simulink model "MCU_LPF_HPF"  (R2021b)
settings: Solver=FixedStepAuto  StartTime=0.0  StopTime=0.03  FixedStep=Ts  RelTol=1e-3
undefined symbols (not defined in the file): f_cutoff
libraries: simulink x1
settings Model: Creator=YeguKang  LastModifiedBy=qorgud1209
settings SFSimCC: SimCustomInitializer=init_software();  SimUserSources=microcontroller.c
settings SFSimCC: SimCustomHeaderCode=|
  | #include "microcontroller.h"
  | #include "Library/Software/headers/Filters.h"
  | #include "Library/Software/headers/ComplexFilters.h"
  | #include "Constants.h"

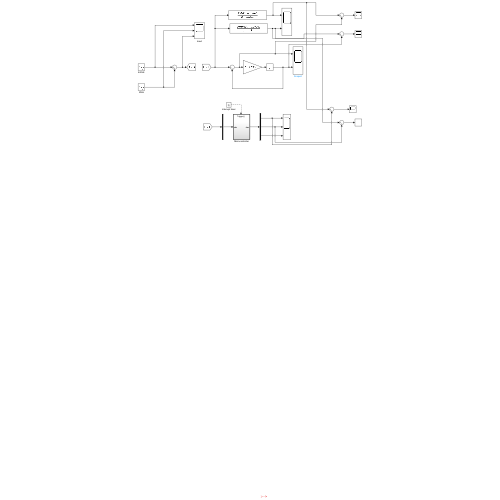
[thumbnail: Simulink's stored preview of the top-level diagram]
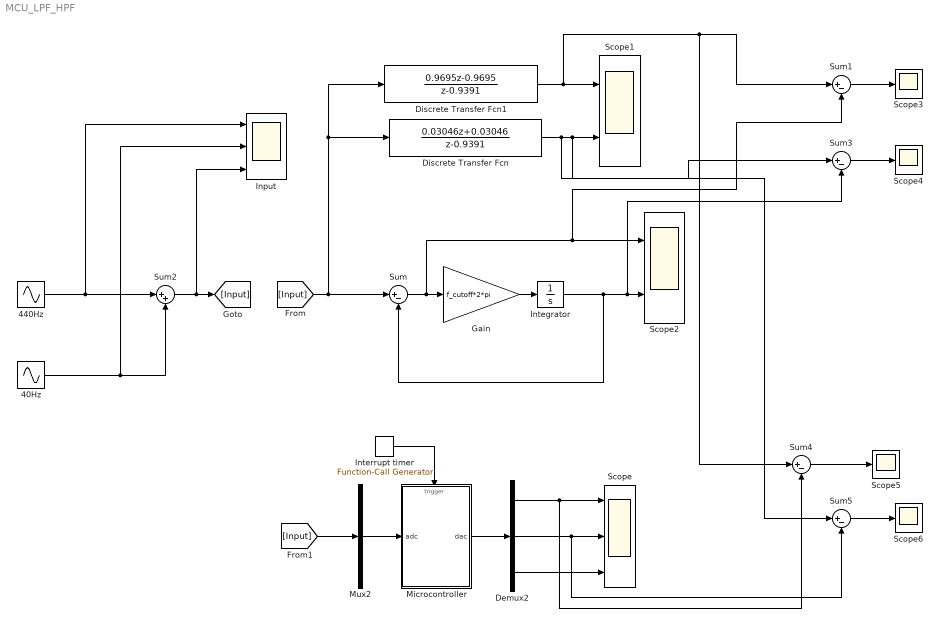
== system MCU_LPF_HPF ==
  40Hz : Sin  Amplitude=2  Frequency=55*2*pi  SampleTime=0
  440Hz : Sin  Frequency=440*(2*pi)  SampleTime=0
  Demux2 : Demux  Outputs=[1 1 1]
  Discrete Transfer Fcn : DiscreteTransferFcn  Numerator=[0.03046 0.03046]  Denominator=[1 -0.9391]
  Discrete Transfer Fcn1 : DiscreteTransferFcn  Numerator=[0.9695 -0.9695]  Denominator=[1 -0.9391]
  Gain : Gain  Gain=f_cutoff*2*pi
  Input : Scope  NumInputPorts=3
  Integrator : Integrator
  Interrupt timer : simulink/Ports & Subsystems/Function-Call Generator  sample_time=Ts  numberOfIterations=1  DisallowWideOutput=off
  Microcontroller : Subsystem
  Mux2 : Mux  Inputs=[1]
  Scope : Scope  NumInputPorts=3
  Scope1 : Scope  NumInputPorts=2
  Scope2 : Scope  NumInputPorts=2
  Scope{3..6} (4 alike) : Scope
  Sum{,1,3..5} (5 alike) : Sum  Inputs=|+-
  Sum2 : Sum  Inputs=|++
  wires:
  Sum/1 -> Sum1/2, Scope2/1, Gain/1
  [Input] -> Discrete Transfer Fcn1/1, Discrete Transfer Fcn/1, Sum/1
  Gain/1 -> Integrator/1
  Interrupt timer/1 -> Microcontroller/Trigger
  Sum2/1 -> Input/3, [Input]
  Mux2/1 -> Microcontroller/1(adc)
  Demux2/2 -> Sum5/2, Scope/2
  [Input] -> Mux2/1
  Demux2/1 -> Sum4/2, Scope/1
  Demux2/3 -> Scope/3
  Integrator/1 -> Sum/2, Sum3/2, Scope2/2
  Microcontroller/1(dac) -> Demux2/1
  440Hz/1 -> Input/1, Sum2/1
  ? -> ?
  40Hz/1 -> Input/2, Sum2/2
  Discrete Transfer Fcn1/1 -> Sum4/1, Sum1/1, Scope1/1
  Discrete Transfer Fcn/1 -> Sum3/1, Sum5/1, Scope1/2
  Sum3/1 -> Scope4/1
  Sum1/1 -> Scope3/1
  Sum4/1 -> Scope5/1
  Sum5/1 -> Scope6/1

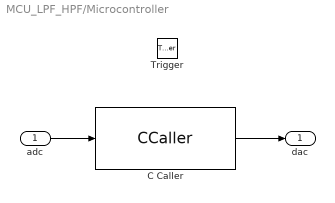
== system MCU_LPF_HPF/Microcontroller ==
  adc : Inport
  Trigger : TriggerPort  TriggerType=function-call  VariantControl=Variant
  C Caller : CCaller  FunctionName=microcontroller  PortSpecificationStruct="%)30     .    N ,   8    (     @         %    \"     (    !     0         %  0 \"0    $    _    07)G3F%M90  4&]R=$YA;64 4V-O<&4     26YD97@     5'EP90      4VEZ90      27-';&]B86P   X    P    !@    @    $          4    (     0    ,    !         !   P!A9&, #@   #     &    \"     0         !0    @    !     P    $         $  # &%D8P .    .     8    (    !          %    \"     $    %     0         0    !0   $EN<'5T    #@   #@    &    \"     8         !0    @    !     0    $         \"0    @               X    X    !@    @    $          4    (     0    8    !         !     &    9&]U8FQE   .    ,     8    (    !          %    \"     $    !     0         0  $ ,0    X    P    !@    @    ) @        4    (     0    $    !          (  0      #@   #     &    \"     0         !0    @    !     P    $         $  # &1A8P .    ,     8    (    !          %    \"     $    #     0         0  , 9&%C  X    X    !@    @    $          4    (     0    8    !         !     &    3W5T<'5T   .    .     8    (    !@         %    \"     $    !     0         )    \"               #@   #@    &    \"     0         !0    @    !    !@    $         $     8   !D;W5B;&4   X    P    !@    @    $          4    (     0    $    !         !   0 S    #@   #     &    \"     D\"        !0    @    !     0    $          @ !"
  dac : Outport  VectorParamsAs1DForOutWhenUnconnected=off
  wires:
  C Caller/1 -> dac/1
  adc/1 -> C Caller/1
